simulink model "Tipo3_v4"  (R2018b)
settings: Solver=FixedStepDiscrete  StartTime=0.0  StopTime=30  MaxStep=50e-6  RelTol=1e-3
PreLoadFcn:
  | Ts=2e-6;
InitFcn:
  | %xInitial = init_power_wind_dfig_det;
  | Ts=2e-6;
undefined symbols (not defined in the file): D1, Delta, DiscIntNeverNeededParam, find_system, level
libraries: powerlib x142, simulink x110, powerlib_meascontrol x63, powerlib_extras x38, simulink_extras x10
(part 4 of 6)

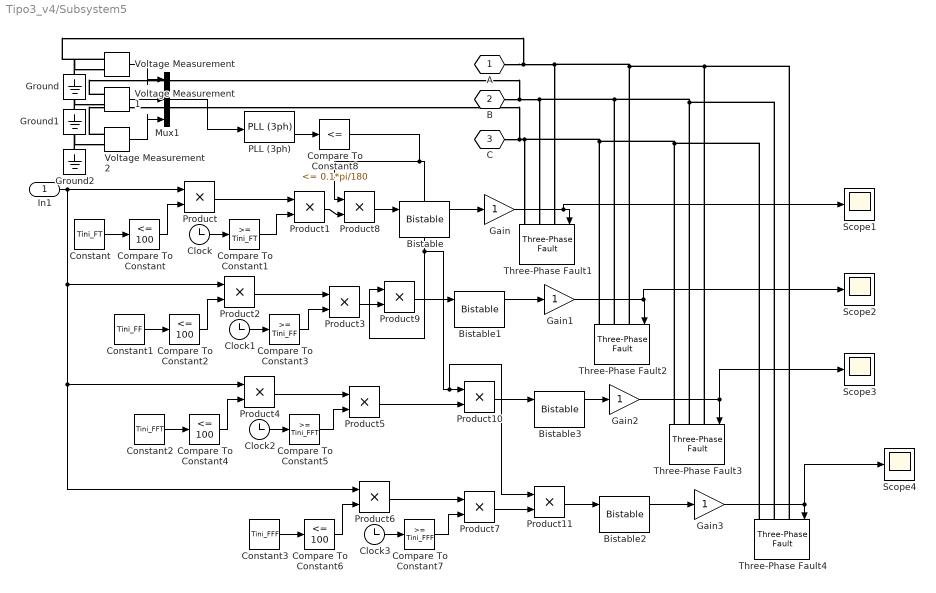
== system Tipo3_v4/Subsystem5 ==
  In1 : Inport
  Bistable{,1..3} (4 alike) : powerlib_meascontrol/Logic/Bistable  Qpriority=Set  ic=0  Ts=Ts
      settings: SourceProductName=Simscape Power Systems  SourceProductBaseCode=PS
  Clock{,1..3} (4 alike) : Clock
  Compare To Constant{,2,4,6} (4 alike) : simulink/Logic and Bit Operations/Compare To Constant  relop=<=  const=100  OutDataTypeStr=uint8
  Compare To Constant1 : simulink/Logic and Bit Operations/Compare To Constant  relop=>=  const=Tini_FT  OutDataTypeStr=uint8
  Compare To Constant3 : simulink/Logic and Bit Operations/Compare To Constant  relop=>=  const=Tini_FF  OutDataTypeStr=uint8
  Compare To Constant5 : simulink/Logic and Bit Operations/Compare To Constant  relop=>=  const=Tini_FFT  OutDataTypeStr=uint8
  Compare To Constant7 : simulink/Logic and Bit Operations/Compare To Constant  relop=>=  const=Tini_FFF  OutDataTypeStr=uint8
  Compare To Constant8 : simulink/Logic and Bit Operations/Compare To Constant  relop=<=  const=0.1*pi/180  OutDataTypeStr=uint8
  Constant : Constant  Value=Tini_FT
  Constant1 : Constant  Value=Tini_FF
  Constant2 : Constant  Value=Tini_FFT
  Constant3 : Constant  Value=Tini_FFF
  Gain{,1..3} (4 alike) : Gain  OutDataTypeStr=double
  Ground : powerlib/Elements/Ground  LConnTagsString=a
  Ground1 : powerlib/Elements/Ground  LConnTagsString=a
  Ground2 : powerlib/Elements/Ground  LConnTagsString=a
  Mux1 : Mux  Inputs=3
  PLL (3ph) : powerlib_meascontrol/PLL/PLL (3ph)  Fmin=60  Par_Init=[0, 60]  ParK=[180, 3200, 1]  TcD=1e-4  MaxRateChangeFreq=12  FilterCutOffFreq=25  Ts=Ts  AGC=on
  Product{,2..7} (7 alike) : Product
  Product{1,8..11} (5 alike) : Product  RndMeth=Ceiling
  Scope{1..4} (4 alike) : Scope
  Three-Phase Fault1 : powerlib/Elements/Three-Phase Fault  InitialStates=0  FaultA=on  FaultB=off  FaultC=off  GroundFault=on  SwitchTimes=[900 1000]  External=on  SwitchStatus=NaN  FaultResistance=R_falta  GroundResistance=R_falta  SnubberResistance=1e6  SnubberCapacitance=inf  Measurements=None
  Three-Phase Fault2 : powerlib/Elements/Three-Phase Fault  InitialStates=0  FaultA=on  FaultB=on  FaultC=off  GroundFault=off  SwitchTimes=[900 1000]  External=on  SwitchStatus=NaN  FaultResistance=R_falta  GroundResistance=1e-12  SnubberResistance=1e6  SnubberCapacitance=inf  Measurements=None
  Three-Phase Fault3 : powerlib/Elements/Three-Phase Fault  InitialStates=0  FaultA=on  FaultB=on  FaultC=off  GroundFault=on  SwitchTimes=[900 1000]  External=on  SwitchStatus=NaN  FaultResistance=R_falta  GroundResistance=R_falta  SnubberResistance=1e6  SnubberCapacitance=inf  Measurements=None
  Three-Phase Fault4 : powerlib/Elements/Three-Phase Fault  InitialStates=0  FaultA=on  FaultB=on  FaultC=on  GroundFault=on  SwitchTimes=[900 1000]  External=on  SwitchStatus=NaN  FaultResistance=R_falta  GroundResistance=R_falta  SnubberResistance=1e6  SnubberCapacitance=inf  Measurements=None
  Voltage Measurement : powerlib/Measurements/Voltage Measurement  PhasorSimulation=off  OutputType=Complex  PSBequivalent=0
  Voltage Measurement1 : powerlib/Measurements/Voltage Measurement  PhasorSimulation=off  OutputType=Complex  PSBequivalent=0
  Voltage Measurement2 : powerlib/Measurements/Voltage Measurement  PhasorSimulation=off  OutputType=Complex  PSBequivalent=0
  A : PMIOPort  Tag=PMCPort  Side=Right
  B : PMIOPort  Tag=PMCPort  Port=2  Side=Right
  C : PMIOPort  Tag=PMCPort  Port=3  Side=Right
  wires:
  Clock/1 -> Compare To Constant1/1
  Product2/1 -> Product3/1
  Constant1/1 -> Compare To Constant2/1
  Product/1 -> Product1/1
  Compare To Constant2/1 -> Product2/2
  Constant2/1 -> Compare To Constant4/1
  Clock2/1 -> Compare To Constant5/1
  Compare To Constant4/1 -> Product4/2
  Clock1/1 -> Compare To Constant3/1
  Compare To Constant5/1 -> Product5/2
  In1/1 -> Product/1, Product2/1, Product4/1, Product6/1
  Clock3/1 -> Compare To Constant7/1
  Constant3/1 -> Compare To Constant6/1
  Compare To Constant6/1 -> Product6/2
  Product6/1 -> Product7/1
  Compare To Constant7/1 -> Product7/2
  Compare To Constant3/1 -> Product3/2
  Constant/1 -> Compare To Constant/1
  Compare To Constant/1 -> Product/2
  Compare To Constant1/1 -> Product1/2
  Product4/1 -> Product5/1
  Product1/1 -> Product8/2
  Product8/1 -> Bistable/1
  Product3/1 -> Product9/2
  Product5/1 -> Product10/2
  Product7/1 -> Product11/2
  Compare To Constant8/1 -> Product11/1, Product10/1, Product9/1, Product8/1
  PLL (3ph)/2 -> Compare To Constant8/1
  Voltage Measurement1/1 -> Mux1/2
  Voltage Measurement/1 -> Mux1/1
  Voltage Measurement2/1 -> Mux1/3
  Mux1/1 -> PLL (3ph)/1
  Gain/1 -> Scope1/1, Three-Phase Fault1/1
  Gain1/1 -> Scope2/1, Three-Phase Fault2/1
  Gain2/1 -> Three-Phase Fault3/1, Scope3/1
  Gain3/1 -> Scope4/1, Three-Phase Fault4/1
  Bistable/1 -> Gain/1
  Product9/1 -> Bistable1/1
  Bistable1/1 -> Gain1/1
  Bistable3/1 -> Gain2/1
  Product10/1 -> Bistable3/1
  Product11/1 -> Bistable2/1
  Bistable2/1 -> Gain3/1
  connections:
  Voltage Measurement1/LConn1 -- B/RConn1 -- Three-Phase Fault1/LConn2 -- Three-Phase Fault2/LConn2 -- Three-Phase Fault3/LConn2 -- Three-Phase Fault4/LConn2
  Voltage Measurement2/LConn1 -- C/RConn1 -- Three-Phase Fault4/LConn3 -- Three-Phase Fault3/LConn3 -- Three-Phase Fault2/LConn3 -- Three-Phase Fault1/LConn3
  A/RConn1 -- Voltage Measurement/LConn1 -- Three-Phase Fault1/LConn1 -- Three-Phase Fault2/LConn1 -- Three-Phase Fault3/LConn1 -- Three-Phase Fault4/LConn1
  Ground/LConn1 -- Voltage Measurement/LConn2
  Ground1/LConn1 -- Voltage Measurement1/LConn2
  Ground2/LConn1 -- Voltage Measurement2/LConn2

== system Tipo3_v4/Subsystem6 ==
  In1 : Inport
  Bistable{,1..3} (4 alike) : powerlib_meascontrol/Logic/Bistable  Qpriority=Set  ic=0  Ts=Ts
      settings: SourceProductName=Simscape Power Systems  SourceProductBaseCode=PS
  Clock{,1..3} (4 alike) : Clock
  Compare To Constant{,2,4,6} (4 alike) : simulink/Logic and Bit Operations/Compare To Constant  relop=<=  const=100  OutDataTypeStr=uint8
  Compare To Constant1 : simulink/Logic and Bit Operations/Compare To Constant  relop=>=  const=Tini_FT  OutDataTypeStr=uint8
  Compare To Constant3 : simulink/Logic and Bit Operations/Compare To Constant  relop=>=  const=Tini_FF  OutDataTypeStr=uint8
  Compare To Constant5 : simulink/Logic and Bit Operations/Compare To Constant  relop=>=  const=Tini_FFT  OutDataTypeStr=uint8
  Compare To Constant7 : simulink/Logic and Bit Operations/Compare To Constant  relop=>=  const=Tini_FFF  OutDataTypeStr=uint8
  Compare To Constant8 : simulink/Logic and Bit Operations/Compare To Constant  relop=<=  const=0.1*pi/180  OutDataTypeStr=uint8
  Constant : Constant  Value=Tini_FT
  Constant1 : Constant  Value=Tini_FF
  Constant2 : Constant  Value=Tini_FFT
  Constant3 : Constant  Value=Tini_FFF
  Gain{,1..3} (4 alike) : Gain  OutDataTypeStr=double
  Ground : powerlib/Elements/Ground  LConnTagsString=a
  Ground1 : powerlib/Elements/Ground  LConnTagsString=a
  Ground2 : powerlib/Elements/Ground  LConnTagsString=a
  Mux1 : Mux  Inputs=3
  PLL (3ph) : powerlib_meascontrol/PLL/PLL (3ph)  Fmin=60  Par_Init=[0, 60]  ParK=[180, 3200, 1]  TcD=1e-4  MaxRateChangeFreq=12  FilterCutOffFreq=25  Ts=Ts  AGC=on
  Product{,2..7} (7 alike) : Product
  Product{1,8..11} (5 alike) : Product  RndMeth=Ceiling
  Scope{1..4} (4 alike) : Scope
  Three-Phase Fault1 : powerlib/Elements/Three-Phase Fault  InitialStates=0  FaultA=on  FaultB=off  FaultC=off  GroundFault=on  SwitchTimes=[900 1000]  External=on  SwitchStatus=NaN  FaultResistance=R_falta  GroundResistance=R_falta  SnubberResistance=1e6  SnubberCapacitance=inf  Measurements=None
  Three-Phase Fault2 : powerlib/Elements/Three-Phase Fault  InitialStates=0  FaultA=on  FaultB=on  FaultC=off  GroundFault=off  SwitchTimes=[900 1000]  External=on  SwitchStatus=NaN  FaultResistance=R_falta  GroundResistance=1e-12  SnubberResistance=1e6  SnubberCapacitance=inf  Measurements=None
  Three-Phase Fault3 : powerlib/Elements/Three-Phase Fault  InitialStates=0  FaultA=on  FaultB=on  FaultC=off  GroundFault=on  SwitchTimes=[900 1000]  External=on  SwitchStatus=NaN  FaultResistance=R_falta  GroundResistance=R_falta  SnubberResistance=1e6  SnubberCapacitance=inf  Measurements=None
  Three-Phase Fault4 : powerlib/Elements/Three-Phase Fault  InitialStates=0  FaultA=on  FaultB=on  FaultC=on  GroundFault=on  SwitchTimes=[900 1000]  External=on  SwitchStatus=NaN  FaultResistance=R_falta  GroundResistance=R_falta  SnubberResistance=1e6  SnubberCapacitance=inf  Measurements=None
  Voltage Measurement : powerlib/Measurements/Voltage Measurement  PhasorSimulation=off  OutputType=Complex  PSBequivalent=0
  Voltage Measurement1 : powerlib/Measurements/Voltage Measurement  PhasorSimulation=off  OutputType=Complex  PSBequivalent=0
  Voltage Measurement2 : powerlib/Measurements/Voltage Measurement  PhasorSimulation=off  OutputType=Complex  PSBequivalent=0
  A : PMIOPort  Tag=PMCPort  Side=Right
  B : PMIOPort  Tag=PMCPort  Port=2  Side=Right
  C : PMIOPort  Tag=PMCPort  Port=3  Side=Right
  wires:
  Clock/1 -> Compare To Constant1/1
  Product2/1 -> Product3/1
  Constant1/1 -> Compare To Constant2/1
  Product/1 -> Product1/1
  Compare To Constant2/1 -> Product2/2
  Constant2/1 -> Compare To Constant4/1
  Clock2/1 -> Compare To Constant5/1
  Compare To Constant4/1 -> Product4/2
  Clock1/1 -> Compare To Constant3/1
  Compare To Constant5/1 -> Product5/2
  In1/1 -> Product/1, Product2/1, Product4/1, Product6/1
  Clock3/1 -> Compare To Constant7/1
  Constant3/1 -> Compare To Constant6/1
  Compare To Constant6/1 -> Product6/2
  Product6/1 -> Product7/1
  Compare To Constant7/1 -> Product7/2
  Compare To Constant3/1 -> Product3/2
  Constant/1 -> Compare To Constant/1
  Compare To Constant/1 -> Product/2
  Compare To Constant1/1 -> Product1/2
  Product4/1 -> Product5/1
  Product1/1 -> Product8/2
  Product8/1 -> Bistable/1
  Product3/1 -> Product9/2
  Product5/1 -> Product10/2
  Product7/1 -> Product11/2
  Compare To Constant8/1 -> Product11/1, Product10/1, Product9/1, Product8/1
  PLL (3ph)/2 -> Compare To Constant8/1
  Voltage Measurement1/1 -> Mux1/2
  Voltage Measurement/1 -> Mux1/1
  Voltage Measurement2/1 -> Mux1/3
  Mux1/1 -> PLL (3ph)/1
  Gain/1 -> Scope1/1, Three-Phase Fault1/1
  Gain1/1 -> Scope2/1, Three-Phase Fault2/1
  Gain2/1 -> Three-Phase Fault3/1, Scope3/1
  Gain3/1 -> Scope4/1, Three-Phase Fault4/1
  Bistable/1 -> Gain/1
  Product9/1 -> Bistable1/1
  Bistable1/1 -> Gain1/1
  Bistable3/1 -> Gain2/1
  Product10/1 -> Bistable3/1
  Product11/1 -> Bistable2/1
  Bistable2/1 -> Gain3/1
  connections:
  Voltage Measurement1/LConn1 -- B/RConn1 -- Three-Phase Fault1/LConn2 -- Three-Phase Fault2/LConn2 -- Three-Phase Fault3/LConn2 -- Three-Phase Fault4/LConn2
  Voltage Measurement2/LConn1 -- C/RConn1 -- Three-Phase Fault4/LConn3 -- Three-Phase Fault3/LConn3 -- Three-Phase Fault2/LConn3 -- Three-Phase Fault1/LConn3
  A/RConn1 -- Voltage Measurement/LConn1 -- Three-Phase Fault1/LConn1 -- Three-Phase Fault2/LConn1 -- Three-Phase Fault3/LConn1 -- Three-Phase Fault4/LConn1
  Ground/LConn1 -- Voltage Measurement/LConn2
  Ground1/LConn1 -- Voltage Measurement1/LConn2
  Ground2/LConn1 -- Voltage Measurement2/LConn2

== system Tipo3_v4/Subsystem7 ==
  In1 : Inport
  Bistable{,1..3} (4 alike) : powerlib_meascontrol/Logic/Bistable  Qpriority=Set  ic=0  Ts=Ts
      settings: SourceProductName=Simscape Power Systems  SourceProductBaseCode=PS
  Clock{,1..3} (4 alike) : Clock
  Compare To Constant{,2,4,6} (4 alike) : simulink/Logic and Bit Operations/Compare To Constant  relop=<=  const=100  OutDataTypeStr=uint8
  Compare To Constant1 : simulink/Logic and Bit Operations/Compare To Constant  relop=>=  const=Tini_FT  OutDataTypeStr=uint8
  Compare To Constant3 : simulink/Logic and Bit Operations/Compare To Constant  relop=>=  const=Tini_FF  OutDataTypeStr=uint8
  Compare To Constant5 : simulink/Logic and Bit Operations/Compare To Constant  relop=>=  const=Tini_FFT  OutDataTypeStr=uint8
  Compare To Constant7 : simulink/Logic and Bit Operations/Compare To Constant  relop=>=  const=Tini_FFF  OutDataTypeStr=uint8
  Compare To Constant8 : simulink/Logic and Bit Operations/Compare To Constant  relop=<=  const=0.1*pi/180  OutDataTypeStr=uint8
  Constant : Constant  Value=Tini_FT
  Constant1 : Constant  Value=Tini_FF
  Constant2 : Constant  Value=Tini_FFT
  Constant3 : Constant  Value=Tini_FFF
  Gain{,1..3} (4 alike) : Gain  OutDataTypeStr=double
  Ground : powerlib/Elements/Ground  LConnTagsString=a
  Ground1 : powerlib/Elements/Ground  LConnTagsString=a
  Ground2 : powerlib/Elements/Ground  LConnTagsString=a
  Mux1 : Mux  Inputs=3
  PLL (3ph) : powerlib_meascontrol/PLL/PLL (3ph)  Fmin=60  Par_Init=[0, 60]  ParK=[180, 3200, 1]  TcD=1e-4  MaxRateChangeFreq=12  FilterCutOffFreq=25  Ts=Ts  AGC=on
  Product{,2..7} (7 alike) : Product
  Product{1,8..11} (5 alike) : Product  RndMeth=Ceiling
  Scope{1..4} (4 alike) : Scope
  Three-Phase Fault1 : powerlib/Elements/Three-Phase Fault  InitialStates=0  FaultA=on  FaultB=off  FaultC=off  GroundFault=on  SwitchTimes=[900 1000]  External=on  SwitchStatus=NaN  FaultResistance=R_falta  GroundResistance=R_falta  SnubberResistance=1e6  SnubberCapacitance=inf  Measurements=None
  Three-Phase Fault2 : powerlib/Elements/Three-Phase Fault  InitialStates=0  FaultA=on  FaultB=on  FaultC=off  GroundFault=off  SwitchTimes=[900 1000]  External=on  SwitchStatus=NaN  FaultResistance=R_falta  GroundResistance=1e-12  SnubberResistance=1e6  SnubberCapacitance=inf  Measurements=None
  Three-Phase Fault3 : powerlib/Elements/Three-Phase Fault  InitialStates=0  FaultA=on  FaultB=on  FaultC=off  GroundFault=on  SwitchTimes=[900 1000]  External=on  SwitchStatus=NaN  FaultResistance=R_falta  GroundResistance=R_falta  SnubberResistance=1e6  SnubberCapacitance=inf  Measurements=None
  Three-Phase Fault4 : powerlib/Elements/Three-Phase Fault  InitialStates=0  FaultA=on  FaultB=on  FaultC=on  GroundFault=on  SwitchTimes=[900 1000]  External=on  SwitchStatus=NaN  FaultResistance=R_falta  GroundResistance=R_falta  SnubberResistance=1e6  SnubberCapacitance=inf  Measurements=None
  Voltage Measurement : powerlib/Measurements/Voltage Measurement  PhasorSimulation=off  OutputType=Complex  PSBequivalent=0
  Voltage Measurement1 : powerlib/Measurements/Voltage Measurement  PhasorSimulation=off  OutputType=Complex  PSBequivalent=0
  Voltage Measurement2 : powerlib/Measurements/Voltage Measurement  PhasorSimulation=off  OutputType=Complex  PSBequivalent=0
  A : PMIOPort  Tag=PMCPort  Side=Right
  B : PMIOPort  Tag=PMCPort  Port=2  Side=Right
  C : PMIOPort  Tag=PMCPort  Port=3  Side=Right
  wires:
  Clock/1 -> Compare To Constant1/1
  Product2/1 -> Product3/1
  Constant1/1 -> Compare To Constant2/1
  Product/1 -> Product1/1
  Compare To Constant2/1 -> Product2/2
  Constant2/1 -> Compare To Constant4/1
  Clock2/1 -> Compare To Constant5/1
  Compare To Constant4/1 -> Product4/2
  Clock1/1 -> Compare To Constant3/1
  Compare To Constant5/1 -> Product5/2
  In1/1 -> Product/1, Product2/1, Product4/1, Product6/1
  Clock3/1 -> Compare To Constant7/1
  Constant3/1 -> Compare To Constant6/1
  Compare To Constant6/1 -> Product6/2
  Product6/1 -> Product7/1
  Compare To Constant7/1 -> Product7/2
  Compare To Constant3/1 -> Product3/2
  Constant/1 -> Compare To Constant/1
  Compare To Constant/1 -> Product/2
  Compare To Constant1/1 -> Product1/2
  Product4/1 -> Product5/1
  Product1/1 -> Product8/2
  Product8/1 -> Bistable/1
  Product3/1 -> Product9/2
  Product5/1 -> Product10/2
  Product7/1 -> Product11/2
  Compare To Constant8/1 -> Product11/1, Product10/1, Product9/1, Product8/1
  PLL (3ph)/2 -> Compare To Constant8/1
  Voltage Measurement1/1 -> Mux1/2
  Voltage Measurement/1 -> Mux1/1
  Voltage Measurement2/1 -> Mux1/3
  Mux1/1 -> PLL (3ph)/1
  Gain/1 -> Scope1/1, Three-Phase Fault1/1
  Gain1/1 -> Scope2/1, Three-Phase Fault2/1
  Gain2/1 -> Three-Phase Fault3/1, Scope3/1
  Gain3/1 -> Scope4/1, Three-Phase Fault4/1
  Bistable/1 -> Gain/1
  Product9/1 -> Bistable1/1
  Bistable1/1 -> Gain1/1
  Bistable3/1 -> Gain2/1
  Product10/1 -> Bistable3/1
  Product11/1 -> Bistable2/1
  Bistable2/1 -> Gain3/1
  connections:
  Voltage Measurement1/LConn1 -- B/RConn1 -- Three-Phase Fault1/LConn2 -- Three-Phase Fault2/LConn2 -- Three-Phase Fault3/LConn2 -- Three-Phase Fault4/LConn2
  Voltage Measurement2/LConn1 -- C/RConn1 -- Three-Phase Fault4/LConn3 -- Three-Phase Fault3/LConn3 -- Three-Phase Fault2/LConn3 -- Three-Phase Fault1/LConn3
  A/RConn1 -- Voltage Measurement/LConn1 -- Three-Phase Fault1/LConn1 -- Three-Phase Fault2/LConn1 -- Three-Phase Fault3/LConn1 -- Three-Phase Fault4/LConn1
  Ground/LConn1 -- Voltage Measurement/LConn2
  Ground1/LConn1 -- Voltage Measurement1/LConn2
  Ground2/LConn1 -- Voltage Measurement2/LConn2

== system Tipo3_v4/Subsystem8 ==
  In1 : Inport
  Bistable{,1..3} (4 alike) : powerlib_meascontrol/Logic/Bistable  Qpriority=Set  ic=0  Ts=Ts
      settings: SourceProductName=Simscape Power Systems  SourceProductBaseCode=PS
  Clock{,1..3} (4 alike) : Clock
  Compare To Constant{,2,4,6} (4 alike) : simulink/Logic and Bit Operations/Compare To Constant  relop=<=  const=100  OutDataTypeStr=uint8
  Compare To Constant1 : simulink/Logic and Bit Operations/Compare To Constant  relop=>=  const=Tini_FT  OutDataTypeStr=uint8
  Compare To Constant3 : simulink/Logic and Bit Operations/Compare To Constant  relop=>=  const=Tini_FF  OutDataTypeStr=uint8
  Compare To Constant5 : simulink/Logic and Bit Operations/Compare To Constant  relop=>=  const=Tini_FFT  OutDataTypeStr=uint8
  Compare To Constant7 : simulink/Logic and Bit Operations/Compare To Constant  relop=>=  const=Tini_FFF  OutDataTypeStr=uint8
  Compare To Constant8 : simulink/Logic and Bit Operations/Compare To Constant  relop=<=  const=0.1*pi/180  OutDataTypeStr=uint8
  Constant : Constant  Value=Tini_FT
  Constant1 : Constant  Value=Tini_FF
  Constant2 : Constant  Value=Tini_FFT
  Constant3 : Constant  Value=Tini_FFF
  Gain{,1..3} (4 alike) : Gain  OutDataTypeStr=double
  Ground : powerlib/Elements/Ground  LConnTagsString=a
  Ground1 : powerlib/Elements/Ground  LConnTagsString=a
  Ground2 : powerlib/Elements/Ground  LConnTagsString=a
  Mux1 : Mux  Inputs=3
  PLL (3ph) : powerlib_meascontrol/PLL/PLL (3ph)  Fmin=60  Par_Init=[0, 60]  ParK=[180, 3200, 1]  TcD=1e-4  MaxRateChangeFreq=12  FilterCutOffFreq=25  Ts=Ts  AGC=on
  Product{,2..7} (7 alike) : Product
  Product{1,8..11} (5 alike) : Product  RndMeth=Ceiling
  Scope{1..4} (4 alike) : Scope
  Three-Phase Fault1 : powerlib/Elements/Three-Phase Fault  InitialStates=0  FaultA=on  FaultB=off  FaultC=off  GroundFault=on  SwitchTimes=[900 1000]  External=on  SwitchStatus=NaN  FaultResistance=R_falta  GroundResistance=R_falta  SnubberResistance=1e6  SnubberCapacitance=inf  Measurements=None
  Three-Phase Fault2 : powerlib/Elements/Three-Phase Fault  InitialStates=0  FaultA=on  FaultB=on  FaultC=off  GroundFault=off  SwitchTimes=[900 1000]  External=on  SwitchStatus=NaN  FaultResistance=R_falta  GroundResistance=1e-12  SnubberResistance=1e6  SnubberCapacitance=inf  Measurements=None
  Three-Phase Fault3 : powerlib/Elements/Three-Phase Fault  InitialStates=0  FaultA=on  FaultB=on  FaultC=off  GroundFault=on  SwitchTimes=[900 1000]  External=on  SwitchStatus=NaN  FaultResistance=R_falta  GroundResistance=R_falta  SnubberResistance=1e6  SnubberCapacitance=inf  Measurements=None
  Three-Phase Fault4 : powerlib/Elements/Three-Phase Fault  InitialStates=0  FaultA=on  FaultB=on  FaultC=on  GroundFault=on  SwitchTimes=[900 1000]  External=on  SwitchStatus=NaN  FaultResistance=R_falta  GroundResistance=R_falta  SnubberResistance=1e6  SnubberCapacitance=inf  Measurements=None
  Voltage Measurement : powerlib/Measurements/Voltage Measurement  PhasorSimulation=off  OutputType=Complex  PSBequivalent=0
  Voltage Measurement1 : powerlib/Measurements/Voltage Measurement  PhasorSimulation=off  OutputType=Complex  PSBequivalent=0
  Voltage Measurement2 : powerlib/Measurements/Voltage Measurement  PhasorSimulation=off  OutputType=Complex  PSBequivalent=0
  A : PMIOPort  Tag=PMCPort  Side=Right
  B : PMIOPort  Tag=PMCPort  Port=2  Side=Right
  C : PMIOPort  Tag=PMCPort  Port=3  Side=Right
  wires:
  Clock/1 -> Compare To Constant1/1
  Product2/1 -> Product3/1
  Constant1/1 -> Compare To Constant2/1
  Product/1 -> Product1/1
  Compare To Constant2/1 -> Product2/2
  Constant2/1 -> Compare To Constant4/1
  Clock2/1 -> Compare To Constant5/1
  Compare To Constant4/1 -> Product4/2
  Clock1/1 -> Compare To Constant3/1
  Compare To Constant5/1 -> Product5/2
  In1/1 -> Product/1, Product2/1, Product4/1, Product6/1
  Clock3/1 -> Compare To Constant7/1
  Constant3/1 -> Compare To Constant6/1
  Compare To Constant6/1 -> Product6/2
  Product6/1 -> Product7/1
  Compare To Constant7/1 -> Product7/2
  Compare To Constant3/1 -> Product3/2
  Constant/1 -> Compare To Constant/1
  Compare To Constant/1 -> Product/2
  Compare To Constant1/1 -> Product1/2
  Product4/1 -> Product5/1
  Product1/1 -> Product8/2
  Product8/1 -> Bistable/1
  Product3/1 -> Product9/2
  Product5/1 -> Product10/2
  Product7/1 -> Product11/2
  Compare To Constant8/1 -> Product11/1, Product10/1, Product9/1, Product8/1
  PLL (3ph)/2 -> Compare To Constant8/1
  Voltage Measurement1/1 -> Mux1/2
  Voltage Measurement/1 -> Mux1/1
  Voltage Measurement2/1 -> Mux1/3
  Mux1/1 -> PLL (3ph)/1
  Gain/1 -> Scope1/1, Three-Phase Fault1/1
  Gain1/1 -> Scope2/1, Three-Phase Fault2/1
  Gain2/1 -> Three-Phase Fault3/1, Scope3/1
  Gain3/1 -> Scope4/1, Three-Phase Fault4/1
  Bistable/1 -> Gain/1
  Product9/1 -> Bistable1/1
  Bistable1/1 -> Gain1/1
  Bistable3/1 -> Gain2/1
  Product10/1 -> Bistable3/1
  Product11/1 -> Bistable2/1
  Bistable2/1 -> Gain3/1
  connections:
  Voltage Measurement1/LConn1 -- B/RConn1 -- Three-Phase Fault1/LConn2 -- Three-Phase Fault2/LConn2 -- Three-Phase Fault3/LConn2 -- Three-Phase Fault4/LConn2
  Voltage Measurement2/LConn1 -- C/RConn1 -- Three-Phase Fault4/LConn3 -- Three-Phase Fault3/LConn3 -- Three-Phase Fault2/LConn3 -- Three-Phase Fault1/LConn3
  A/RConn1 -- Voltage Measurement/LConn1 -- Three-Phase Fault1/LConn1 -- Three-Phase Fault2/LConn1 -- Three-Phase Fault3/LConn1 -- Three-Phase Fault4/LConn1
  Ground/LConn1 -- Voltage Measurement/LConn2
  Ground1/LConn1 -- Voltage Measurement1/LConn2
  Ground2/LConn1 -- Voltage Measurement2/LConn2

== system Tipo3_v4/Subsystem9 ==
  In1 : Inport
  Bistable{,1..3} (4 alike) : powerlib_meascontrol/Logic/Bistable  Qpriority=Set  ic=0  Ts=Ts
      settings: SourceProductName=Simscape Power Systems  SourceProductBaseCode=PS
  Clock{,1..3} (4 alike) : Clock
  Compare To Constant{,2,4,6} (4 alike) : simulink/Logic and Bit Operations/Compare To Constant  relop=<=  const=100  OutDataTypeStr=uint8
  Compare To Constant1 : simulink/Logic and Bit Operations/Compare To Constant  relop=>=  const=Tini_FT  OutDataTypeStr=uint8
  Compare To Constant3 : simulink/Logic and Bit Operations/Compare To Constant  relop=>=  const=Tini_FF  OutDataTypeStr=uint8
  Compare To Constant5 : simulink/Logic and Bit Operations/Compare To Constant  relop=>=  const=Tini_FFT  OutDataTypeStr=uint8
  Compare To Constant7 : simulink/Logic and Bit Operations/Compare To Constant  relop=>=  const=Tini_FFF  OutDataTypeStr=uint8
  Compare To Constant8 : simulink/Logic and Bit Operations/Compare To Constant  relop=<=  const=0.1*pi/180  OutDataTypeStr=uint8
  Constant : Constant  Value=Tini_FT
  Constant1 : Constant  Value=Tini_FF
  Constant2 : Constant  Value=Tini_FFT
  Constant3 : Constant  Value=Tini_FFF
  Gain{,1..3} (4 alike) : Gain  OutDataTypeStr=double
  Ground : powerlib/Elements/Ground  LConnTagsString=a
  Ground1 : powerlib/Elements/Ground  LConnTagsString=a
  Ground2 : powerlib/Elements/Ground  LConnTagsString=a
  Mux1 : Mux  Inputs=3
  PLL (3ph) : powerlib_meascontrol/PLL/PLL (3ph)  Fmin=60  Par_Init=[0, 60]  ParK=[180, 3200, 1]  TcD=1e-4  MaxRateChangeFreq=12  FilterCutOffFreq=25  Ts=Ts  AGC=on
  Product{,2..7} (7 alike) : Product
  Product{1,8..11} (5 alike) : Product  RndMeth=Ceiling
  Scope{1..4} (4 alike) : Scope
  Three-Phase Fault1 : powerlib/Elements/Three-Phase Fault  InitialStates=0  FaultA=on  FaultB=off  FaultC=off  GroundFault=on  SwitchTimes=[900 1000]  External=on  SwitchStatus=NaN  FaultResistance=R_falta  GroundResistance=R_falta  SnubberResistance=1e6  SnubberCapacitance=inf  Measurements=None
  Three-Phase Fault2 : powerlib/Elements/Three-Phase Fault  InitialStates=0  FaultA=on  FaultB=on  FaultC=off  GroundFault=off  SwitchTimes=[900 1000]  External=on  SwitchStatus=NaN  FaultResistance=R_falta  GroundResistance=1e-12  SnubberResistance=1e6  SnubberCapacitance=inf  Measurements=None
  Three-Phase Fault3 : powerlib/Elements/Three-Phase Fault  InitialStates=0  FaultA=on  FaultB=on  FaultC=off  GroundFault=on  SwitchTimes=[900 1000]  External=on  SwitchStatus=NaN  FaultResistance=R_falta  GroundResistance=R_falta  SnubberResistance=1e6  SnubberCapacitance=inf  Measurements=None
  Three-Phase Fault4 : powerlib/Elements/Three-Phase Fault  InitialStates=0  FaultA=on  FaultB=on  FaultC=on  GroundFault=on  SwitchTimes=[900 1000]  External=on  SwitchStatus=NaN  FaultResistance=R_falta  GroundResistance=R_falta  SnubberResistance=1e6  SnubberCapacitance=inf  Measurements=None
  Voltage Measurement : powerlib/Measurements/Voltage Measurement  PhasorSimulation=off  OutputType=Complex  PSBequivalent=0
  Voltage Measurement1 : powerlib/Measurements/Voltage Measurement  PhasorSimulation=off  OutputType=Complex  PSBequivalent=0
  Voltage Measurement2 : powerlib/Measurements/Voltage Measurement  PhasorSimulation=off  OutputType=Complex  PSBequivalent=0
  A : PMIOPort  Tag=PMCPort  Side=Right
  B : PMIOPort  Tag=PMCPort  Port=2  Side=Right
  C : PMIOPort  Tag=PMCPort  Port=3  Side=Right
  wires:
  Clock/1 -> Compare To Constant1/1
  Product2/1 -> Product3/1
  Constant1/1 -> Compare To Constant2/1
  Product/1 -> Product1/1
  Compare To Constant2/1 -> Product2/2
  Constant2/1 -> Compare To Constant4/1
  Clock2/1 -> Compare To Constant5/1
  Compare To Constant4/1 -> Product4/2
  Clock1/1 -> Compare To Constant3/1
  Compare To Constant5/1 -> Product5/2
  In1/1 -> Product/1, Product2/1, Product4/1, Product6/1
  Clock3/1 -> Compare To Constant7/1
  Constant3/1 -> Compare To Constant6/1
  Compare To Constant6/1 -> Product6/2
  Product6/1 -> Product7/1
  Compare To Constant7/1 -> Product7/2
  Compare To Constant3/1 -> Product3/2
  Constant/1 -> Compare To Constant/1
  Compare To Constant/1 -> Product/2
  Compare To Constant1/1 -> Product1/2
  Product4/1 -> Product5/1
  Product1/1 -> Product8/2
  Product8/1 -> Bistable/1
  Product3/1 -> Product9/2
  Product5/1 -> Product10/2
  Product7/1 -> Product11/2
  Compare To Constant8/1 -> Product11/1, Product10/1, Product9/1, Product8/1
  PLL (3ph)/2 -> Compare To Constant8/1
  Voltage Measurement1/1 -> Mux1/2
  Voltage Measurement/1 -> Mux1/1
  Voltage Measurement2/1 -> Mux1/3
  Mux1/1 -> PLL (3ph)/1
  Gain/1 -> Scope1/1, Three-Phase Fault1/1
  Gain1/1 -> Scope2/1, Three-Phase Fault2/1
  Gain2/1 -> Three-Phase Fault3/1, Scope3/1
  Gain3/1 -> Scope4/1, Three-Phase Fault4/1
  Bistable/1 -> Gain/1
  Product9/1 -> Bistable1/1
  Bistable1/1 -> Gain1/1
  Bistable3/1 -> Gain2/1
  Product10/1 -> Bistable3/1
  Product11/1 -> Bistable2/1
  Bistable2/1 -> Gain3/1
  connections:
  Voltage Measurement1/LConn1 -- B/RConn1 -- Three-Phase Fault1/LConn2 -- Three-Phase Fault2/LConn2 -- Three-Phase Fault3/LConn2 -- Three-Phase Fault4/LConn2
  Voltage Measurement2/LConn1 -- C/RConn1 -- Three-Phase Fault4/LConn3 -- Three-Phase Fault3/LConn3 -- Three-Phase Fault2/LConn3 -- Three-Phase Fault1/LConn3
  A/RConn1 -- Voltage Measurement/LConn1 -- Three-Phase Fault1/LConn1 -- Three-Phase Fault2/LConn1 -- Three-Phase Fault3/LConn1 -- Three-Phase Fault4/LConn1
  Ground/LConn1 -- Voltage Measurement/LConn2
  Ground1/LConn1 -- Voltage Measurement1/LConn2
  Ground2/LConn1 -- Voltage Measurement2/LConn2

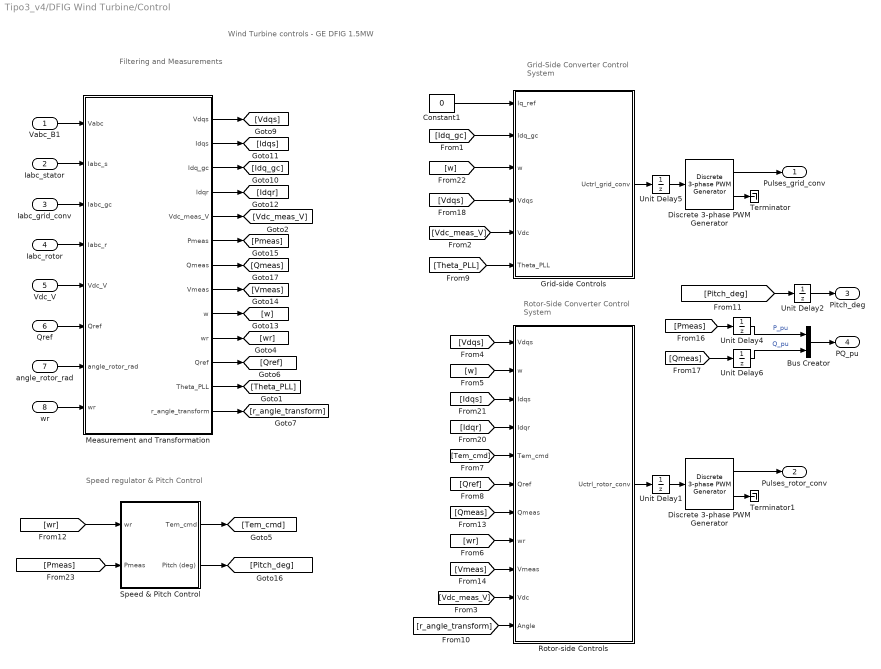
== system Tipo3_v4/DFIG Wind Turbine/Control ==
  note: Speed regulator & Pitch Control
  note: Grid-Side Converter
      | Control System
  note: Rotor-Side Converter
      | Control System
  note: Filtering and
      | Measurements
  note: Wind Turbine controls - GE DFIG 1.5MW
  Vabc_B1 : Inport
  Iabc_stator : Inport  Port=2
  Iabc_grid_conv : Inport  Port=3
  Iabc_rotor : Inport  Port=4
  Vdc_V : Inport  Port=5
  Qref : Inport  Port=6
  angle_rotor_rad : Inport  Port=7
  wr : Inport  Port=8
  Bus Creator : BusCreator  Inputs=2
  Constant1 : Constant  Value=0
  Discrete 3-phase PWM Generator : powerlib_extras/Discrete  Control Blocks/Discrete 3-phase PWM Generator  ModulatorType=2-level  ModulatorMode=Un-synchronized  nF=27  Fc=PWM_freq_grid  ModulatingSignals=off  m=0.2  Freq=60  Phase=0  Ts=Ts
  "Discrete 3-phase PWM Generator " : powerlib_extras/Discrete  Control Blocks/Discrete 3-phase PWM Generator  ModulatorType=2-level  ModulatorMode=Un-synchronized  nF=27  Fc=PWM_freq_rotor  ModulatingSignals=off  m=0.2  Freq=60  Phase=0  Ts=Ts
  Grid-side Controls : Subsystem
  Measurement and Transformation : Subsystem
  Rotor-side Controls : Subsystem
  Speed & Pitch Control : Subsystem
  Terminator : Terminator
  Terminator1 : Terminator
  Unit Delay{1..2,4..6} (5 alike) : UnitDelay  SampleTime=Ts
  Pulses_grid_conv : Outport
  Pulses_rotor_conv : Outport  Port=2
  Pitch_deg : Outport  Port=3
  PQ_pu : Outport  Port=4
  wires:
  Unit Delay6/1 -> Bus Creator/2  "Q_pu"
  Unit Delay4/1 -> Bus Creator/1  "P_pu"
  Unit Delay2/1 -> Pitch_deg/1
  Unit Delay1/1 -> "Discrete 3-phase PWM Generator "/1
  Unit Delay5/1 -> Discrete 3-phase PWM Generator/1
  "Discrete 3-phase PWM Generator "/2 -> Terminator1/1
  Discrete 3-phase PWM Generator/2 -> Terminator/1
  "Discrete 3-phase PWM Generator "/1 -> Pulses_rotor_conv/1
  Discrete 3-phase PWM Generator/1 -> Pulses_grid_conv/1
  Rotor-side Controls/1(Uctrl_rotor_conv) -> Unit Delay1/1
  Grid-side Controls/1(Uctrl_grid_conv) -> Unit Delay5/1
  [Qmeas] -> Unit Delay6/1
  [Pmeas] -> Unit Delay4/1
  Bus Creator/1 -> PQ_pu/1
  Speed & Pitch Control/1(Tem_cmd) -> [Tem_cmd]
  Speed & Pitch Control/2(Pitch (deg)) -> [Pitch_deg]
  [r_angle_transform] -> Rotor-side Controls/11(Angle)
  [Vdc_meas_V] -> Rotor-side Controls/10(Vdc)
  Measurement and Transformation/13(r_angle_transform) -> [r_angle_transform]
  [Theta_PLL] -> Grid-side Controls/6(Theta_PLL)
  Measurement and Transformation/12(Theta_PLL) -> [Theta_PLL]
  [Vmeas] -> Rotor-side Controls/9(Vmeas)
  Measurement and Transformation/8(Vmeas) -> [Vmeas]
  [Qmeas] -> Rotor-side Controls/7(Qmeas)
  Measurement and Transformation/7(Qmeas) -> [Qmeas]
  Vabc_B1/1 -> Measurement and Transformation/1(Vabc)
  Iabc_grid_conv/1 -> Measurement and Transformation/3(Iabc_gc)
  Iabc_rotor/1 -> Measurement and Transformation/4(Iabc_r)
  Iabc_stator/1 -> Measurement and Transformation/2(Iabc_s)
  angle_rotor_rad/1 -> Measurement and Transformation/7(angle_rotor_rad)
  Constant1/1 -> Grid-side Controls/1(Iq_ref)
  Measurement and Transformation/1(Vdqs) -> [Vdqs]
  Measurement and Transformation/2(Idqs) -> [Idqs]
  Measurement and Transformation/3(Idq_gc) -> [Idq_gc]
  Measurement and Transformation/4(Idqr) -> [Idqr]
  Measurement and Transformation/6(Pmeas) -> [Pmeas]
  Measurement and Transformation/9(w) -> [w]
  [Idq_gc] -> Grid-side Controls/2(Idq_gc)
  [w] -> Grid-side Controls/3(w)
  [Vdqs] -> Grid-side Controls/4(Vdqs)
  [Vdc_meas_V] -> Grid-side Controls/5(Vdc)
  [Vdqs] -> Rotor-side Controls/1(Vdqs)
  [w] -> Rotor-side Controls/2(w)
  [Idqs] -> Rotor-side Controls/3(Idqs)
  [Idqr] -> Rotor-side Controls/4(Idqr)
  [Tem_cmd] -> Rotor-side Controls/5(Tem_cmd)
  [Qref] -> Rotor-side Controls/6(Qref)
  [wr] -> Speed & Pitch Control/1(wr)
  Measurement and Transformation/5(Vdc_meas_V) -> [Vdc_meas_V]
  Measurement and Transformation/10("wr ") -> [wr]
  Measurement and Transformation/11("Qref ") -> [Qref]
  Vdc_V/1 -> Measurement and Transformation/5(Vdc_V)
  Qref/1 -> Measurement and Transformation/6(Qref)
  wr/1 -> Measurement and Transformation/8(wr)
  [Pmeas] -> Speed & Pitch Control/2(Pmeas)
  [Pitch_deg] -> Unit Delay2/1
  [wr] -> Rotor-side Controls/8(wr)

== system Tipo3_v4/DFIG Wind Turbine/Drive Train ==
  note: Shaft
  note: Turbine
  note: Wind turbine drive train based on a 2-masse model
  T_wt (pu) : Inport
  Generator speed (pu) : Inport  Port=2
  1_2H_WT : Gain  Gain=1/(2*H_WT)  SaturateOnIntegerOverflow=on  OutDataTypeStr=Inherit: Same as input  ParamDataTypeStr=Inherit: Same as input
  Discrete-Time Integrator : DiscreteIntegrator  InitialCondition=w_wt0  SampleTime=Ts  ICPrevOutput=DiscIntNeverNeededParam  ICPrevScaledInput=DiscIntNeverNeededParam
  Discrete-Time Integrator1 : DiscreteIntegrator  InitialCondition=torque0/Ksh  SampleTime=Ts  ICPrevOutput=DiscIntNeverNeededParam  ICPrevScaledInput=DiscIntNeverNeededParam
  Mutual damping : Gain  Gain=D_mutual  SaturateOnIntegerOverflow=on  OutDataTypeStr=Inherit: Same as input  ParamDataTypeStr=Inherit: Same as input
  Stiffness : Gain  Gain=Ksh  SaturateOnIntegerOverflow=on  OutDataTypeStr=Inherit: Same as input  ParamDataTypeStr=Inherit: Same as input
  Sum : Sum  Inputs=+-  SaturateOnIntegerOverflow=on  InputSameDT=on  OutDataTypeStr=Inherit: Same as first input
  Sum1 : Sum  Inputs=+-  SaturateOnIntegerOverflow=on  InputSameDT=on  OutDataTypeStr=Inherit: Same as first input
  Sum2 : Sum  SaturateOnIntegerOverflow=on  InputSameDT=on  OutDataTypeStr=Inherit: Same as first input
  wbase : Gain  Gain=wbase  SaturateOnIntegerOverflow=on  OutDataTypeStr=Inherit: Same as input  ParamDataTypeStr=Inherit: Same as input
  W_wt (pu) : Outport
  T_shaft (pu) : Outport  Port=2
  wires:
  wbase/1 -> Discrete-Time Integrator1/1
  Discrete-Time Integrator1/1 -> Stiffness/1
  Stiffness/1 -> Sum2/1
  Sum/1 -> 1_2H_WT/1
  1_2H_WT/1 -> Discrete-Time Integrator/1
  Discrete-Time Integrator/1 -> Sum1/1, W_wt (pu)/1
  Generator speed (pu)/1 -> Sum1/2
  Sum1/1 -> wbase/1, Mutual damping/1
  Mutual damping/1 -> Sum2/2
  Sum2/1 -> Sum/2, T_shaft (pu)/1
  T_wt (pu)/1 -> Sum/1

== system Tipo3_v4/DFIG Wind Turbine/Wind Turbine ==
  W_wt (pu) : Inport
  Pitch angle (deg) : Inport  Port=2
  Wind speed (m/s) : Inport  Port=3
  ->pu : Gain  Gain=1/Prated
  Avoid div. by zero : Saturate  UpperLimit=inf  LowerLimit=eps
  "Avoid div. by zero " : Saturate  UpperLimit=inf  LowerLimit=eps
  Fcn1 : Fcn  Expr=K1*u[2]/u[1]
  Fcn2 : Fcn  Expr=c1*(c6*u[1] + (-c4 - c3*(2.5 + u[2]) + c2*(1/(u[1] + c7*(2.5 + u[2])) -c8/(1 + (2.5 + u[2])^3)))/exp(c5*(1/(u[1] + c7*(2.5 + u[2])) - c8/(1 + (2.5 + u[2])^3))))
  "K2*Cp*wind^3 " : Fcn  Expr=K2*u[1]^3*u[2]
  Mux : Mux  Inputs=2
  Mux1 : Mux  Inputs=2
  Mux2 : Mux  Inputs=2
  Product2 : Product  Inputs=*/  SaturateOnIntegerOverflow=on  InputSameDT=on  OutDataTypeStr=Inherit: Same as first input
  Tt (pu) : Outport
  wires:
  "K2*Cp*wind^3 "/1 -> ->pu/1
  "Avoid div. by zero "/1 -> Product2/2, Mux/2
  Avoid div. by zero/1 -> Mux/1, Mux2/1
  W_wt (pu)/1 -> "Avoid div. by zero "/1
  Pitch angle (deg)/1 -> Mux1/2
  Mux2/1 -> "K2*Cp*wind^3 "/1
  Fcn2/1 -> Mux2/2  "Cp"
  Mux/1 -> Fcn1/1
  Mux1/1 -> Fcn2/1
  Fcn1/1 -> Mux1/1  "lambda"
  Wind speed (m/s)/1 -> Avoid div. by zero/1
  Product2/1 -> Tt (pu)/1
  ->pu/1 -> Product2/1  "power_pu"

== system Tipo3_v4/DFIG Wind Turbine/Control/Grid-side Controls ==
  note: Uctrl grid converter
  note: Modulation index & phase
  note: Current regulator
  note: Vdc regulator
  note: Required value for modulation index "m" to obtain 1 pu generated voltage by the converter:
  note: m = Vnom * 2*sqrt(2/3) / Vdc
  note: Where Vnom = RMS ph-ph nominal voltage
  note: Wind Turbine controls - Grid-side converter control system
  Iq_ref : Inport
  Idq_gc : Inport  Port=2
  w : Inport  Port=3
  Vdqs : Inport  Port=4
  Vdc : Inport  Port=5
  Theta_PLL : Inport  Port=6
  ->pu : Gain  Gain=1/Vdc_nom
  0-Mod_index_max_grid : Saturate  UpperLimit=Mod_index_max_grid  LowerLimit=0
  Avoid division by zero : Saturate  UpperLimit=inf  LowerLimit=1e-6
  Cartesian to Polar1 : simulink_extras/Transformations/Cartesian to Polar
      settings: SourceProductName=Simulink
  Constant1 : Constant  Value=L_RL
  Constant2 : Constant  Value=L_RL
  Constant3 : Constant  Value=R_RL
  Constant4 : Constant  Value=R_RL
  Demux{,1..3} (4 alike) : Demux  Outputs=2
  Discrete PI Controller : powerlib_extras/Discrete  Control Blocks/Discrete PI Controller  Kp=Kp_dc  Ki=Ki_dc  Par_Limits=[1 -1]*Imax_grid_conv  Init=0  Ts=Ts
  Discrete PI Controller1 : powerlib_extras/Discrete  Control Blocks/Discrete PI Controller  Kp=Kp_grid_side_cur_reg  Ki=Ki_grid_side_cur_reg  Par_Limits=[1.0 -1.0] *Lim_grid_side_cur_reg  Init=0  Ts=Ts
  K : Constant  Value=Vnom*2*sqrt(2/3)
  Mux : Mux  Inputs=2
  Mux2 : Mux  Inputs=2
  Mux4 : Mux  Inputs=3
  Mux5 : Mux  Inputs=2
  Polar to Cartesian : simulink_extras/Transformations/Polar to Cartesian
      settings: SourceProductName=Simulink  SourceProductBaseCode=SL
  Product : Product  Inputs=3  SaturateOnIntegerOverflow=on  InputSameDT=on  OutDataTypeStr=Inherit: Same as first input
  Product1 : Product  Inputs=3  SaturateOnIntegerOverflow=on  InputSameDT=on  OutDataTypeStr=Inherit: Same as first input
  Product2 : Product  SaturateOnIntegerOverflow=on  InputSameDT=on  OutDataTypeStr=Inherit: Same as first input
  Product3 : Product  SaturateOnIntegerOverflow=on  InputSameDT=on  OutDataTypeStr=Inherit: Same as first input
  Product4 : Product  Inputs=**/  SaturateOnIntegerOverflow=on  InputSameDT=on  OutDataTypeStr=Inherit: Same as first input
  Sum1 : Sum  Inputs=+-  SaturateOnIntegerOverflow=on  InputSameDT=on  OutDataTypeStr=Inherit: Same as first input
  Sum2 : Sum  Inputs=-+|  SaturateOnIntegerOverflow=on  InputSameDT=on  OutDataTypeStr=Inherit: Same as first input
  Sum3 : Sum  Inputs=||++-  SaturateOnIntegerOverflow=on  InputSameDT=on  OutDataTypeStr=Inherit: Same as first input
  Sum4 : Sum  Inputs=|+-  SaturateOnIntegerOverflow=on  InputSameDT=on  OutDataTypeStr=Inherit: Same as first input
  Sum5 : Sum  Inputs=|--+  SaturateOnIntegerOverflow=on  InputSameDT=on  OutDataTypeStr=Inherit: Same as first input
  Sum6 : Sum  Inputs=|-+  SaturateOnIntegerOverflow=on  InputSameDT=on  OutDataTypeStr=Inherit: Same as first input
  Sum7 : Sum  Inputs=|+-  SaturateOnIntegerOverflow=on  InputSameDT=on  OutDataTypeStr=Inherit: Same as first input
  Trigonometric Function2 : Trigonometry
  Trigonometric Function3 : Trigonometry  Operator=cos
  V0 : Constant  Value=0
  Vdc_ref (V) : Constant  Value=Vdc_nom
  dq0_to_abc Transformation : powerlib_extras/Measurements/dq0_to_abc Transformation
  Uctrl_grid_conv : Outport
  wires:
  Sum6/1 -> Cartesian to Polar1/2  "Vq_ctrl_grid_conv"
  Sum1/1 -> Cartesian to Polar1/1  "Vd_ctrl_grid_conv"
  dq0_to_abc Transformation/1 -> Uctrl_grid_conv/1
  Theta_PLL/1 -> Trigonometric Function2/1, Trigonometric Function3/1
  Mux4/1 -> dq0_to_abc Transformation/1  "Vdq0"
  Polar to Cartesian/2 -> Mux4/2
  Polar to Cartesian/1 -> Mux4/1
  V0/1 -> Mux4/3
  Trigonometric Function3/1 -> Mux5/2
  Trigonometric Function2/1 -> Mux5/1
  Mux5/1 -> dq0_to_abc Transformation/2
  [Vdc] -> Avoid division by zero/1
  Product4/1 -> 0-Mod_index_max_grid/1  "m"
  K/1 -> Product4/2
  Avoid division by zero/1 -> Product4/3
  Cartesian to Polar1/1 -> Product4/1
  0-Mod_index_max_grid/1 -> Polar to Cartesian/1
  Cartesian to Polar1/2 -> Polar to Cartesian/2
  Mux/1 -> Demux1/1
  Idq_gc/1 -> Demux/1
  w/1 -> [w]
  Constant2/1 -> Product1/2
  Discrete PI Controller1/1 -> Demux3/1
  Mux2/1 -> Discrete PI Controller1/1
  Demux2/1 -> Sum3/1  "Vd"
  Constant1/1 -> Product/1
  Vdqs/1 -> Demux2/1
  Demux/2 -> Sum2/1  "Iq"
  Demux/1 -> Sum4/2  "Id"
  Product/1 -> Sum3/2
  Constant3/1 -> Product2/1
  Constant4/1 -> Product3/2
  Product1/1 -> Sum5/2
  Demux2/2 -> Sum5/3  "Vq"
  Product2/1 -> Sum3/3
  Product3/1 -> Sum5/1
  Sum4/1 -> Mux2/1
  Sum2/1 -> Mux2/2
  [w] -> Product1/3
  [w] -> Product/2
  [iq_ref] -> Product/3
  [id_ref] -> Product2/2
  [iq_ref] -> Product3/1
  [id_ref] -> Product1/1
  Demux3/1 -> Sum1/2  "vd'"
  Demux3/2 -> Sum6/1  "vq'"
  Demux1/2 -> [iq_ref], Sum2/2  "Iq_ref"
  Demux1/1 -> Sum4/1, [id_ref]  "Id_ref"
  Sum3/1 -> Sum1/1
  Sum5/1 -> Sum6/2
  Discrete PI Controller/1 -> Mux/1  "Id_ref"
  Sum7/1 -> ->pu/1
  ->pu/1 -> Discrete PI Controller/1
  Vdc/1 -> [Vdc], Sum7/2
  Iq_ref/1 -> Mux/2  "Iq_ref"
  Vdc_ref (V)/1 -> Sum7/1
